simulink model "mpc1"  (R2018a)
settings: Solver=FixedStepAuto  StartTime=0.0  StopTime=inf  RelTol=1e-3  EnableMultiTasking=on
libraries: arduinolib x4, simulink x2, mpclib x1
settings Model: SimulationMode=external  ExtModeTrigDuration=2  Creator=stayn  LastModifiedBy=stayn
settings OptimizationCC: EnhancedBackFolding=on  PassReuseOutputArgsAs=Individual arguments  MaxStackSize=64  OptimizeBlockOrder=speed  DifferentSizesBufferReuse=on  OptimizationCustomize=off
settings DebuggingCC: ParameterTunabilityLossMsg=error
settings HardwareCC: ProdBitPerInt=16  ProdBitPerPointer=16  ProdBitPerSizeT=16  ProdBitPerPtrDiffT=16  ProdLargestAtomicFloat=None  ProdWordSize=8  ProdHWDeviceType=Atmel->AVR
settings SFSimCC: MATLABDynamicMemAlloc=off
settings RTWCC: SystemTargetFile=ert.tlc  HardwareBoard=Arduino Mega 2560  TLCOptions=-aInlineSetEventsForThisBaseRateFcn=TLC_FALSE -aSuppressMultiTaskScheduler=TLC_FALSE -aRateBasedStepFcn=1  TemplateMakefile=ert_default_tmf  GenerateReport=on  Toolchain=Arduino AVR  BuildConfiguration=Faster Runs  IncludeHyperlinkInReport=on  LaunchReport=on  GenerateTraceInfo=on  GenerateTraceReport=on  GenerateTraceReportSl=on  GenerateTraceReportSf=on  GenerateTraceReportEml=on
settings CodeAppCC: ForceParamTrailComments=on  IgnoreCustomStorageClasses=off  OperatorAnnotations=on  SimulinkDataObjDesc=on  SFDataObjDesc=on  InsertBlockDesc=on
settings ERTTargetCC: SupportContinuousTime=on  SupportVariableSizeSignals=on

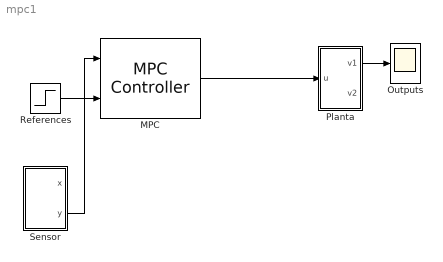
== system mpc1 ==
  MPC : mpclib/MPC Controller  SCDEnableBlockLinearizationSpecification=on  mpcobj=mpc1_C  is_multiple=0  enable_value=0  return_u0=off  updateMPCinCallerWorkspace=on  ref_from_ws=off  ref_signal_name=[]  ref_preview=off  md_from_ws=off  md_signal_name=[]  md_preview=off  from_project=off  project_file=MPCtask.mat  md_inport=off  mv_inport=off  cost_outport=off  return_sequence=off  return_qpstatus=off  return_state=off  state_inport=off  lims_inport=off  cc_inport=off  ywt_inport=off  is_designfromscratch=0  uwt_inport=off  duwt_inport=off  rhoeps_inport=off  uref_inport=off  n_ts=0.1  n_p=10  n_mv=2  n_md=0  n_ud=0  n_mo=2  n_uo=0  BlockDataType=double  SampleTimeInherited=off  switch_inport=off
  Outputs : Scope
  Planta : Subsystem
  References : Step  Before=[0;0]  After=[1;0]
  Sensor : Subsystem
  wires:
  References/1 -> MPC/2
  Planta/1(v1) -> Outputs/1
  MPC/1 -> Planta/1(u)
  Sensor/2(y) -> MPC/1

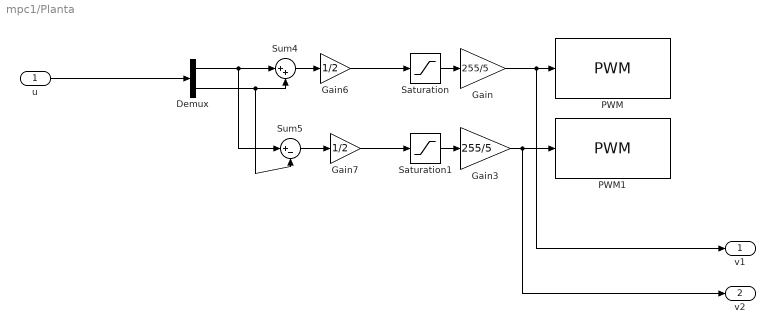
== system mpc1/Planta ==
  u : Inport
  Demux : Demux  Outputs=2
  Gain : Gain  Gain=255/5
  Gain3 : Gain  Gain=255/5
  Gain6 : Gain  Gain=1/2
  Gain7 : Gain  Gain=1/2
  PWM : arduinolib/PWM  pinNumber=9  EnableInputFrequency=off  InitialFrequency=2000  InitialDutyCycle=0  NotificationType=None  blockPlatform=arduino
  PWM1 : arduinolib/PWM  pinNumber=8  EnableInputFrequency=off  InitialFrequency=2000  InitialDutyCycle=0  NotificationType=None  blockPlatform=arduino
  Saturation : Saturate  UpperLimit=5  LowerLimit=0
  Saturation1 : Saturate  UpperLimit=5  LowerLimit=0
  Sum4 : Sum  Inputs=|++
  Sum5 : Sum  Inputs=|+-
  v1 : Outport
  "v2 " : Outport  Port=2
  wires:
  Sum4/1 -> Gain6/1
  Demux/1 -> Sum5/1, Sum4/1
  Saturation1/1 -> Gain3/1
  Gain7/1 -> Saturation1/1
  Demux/2 -> Sum5/2, Sum4/2
  Gain/1 -> PWM/1, v1/1
  Saturation/1 -> Gain/1
  Gain6/1 -> Saturation/1
  Gain3/1 -> PWM1/1, "v2 "/1
  Sum5/1 -> Gain7/1
  u/1 -> Demux/1

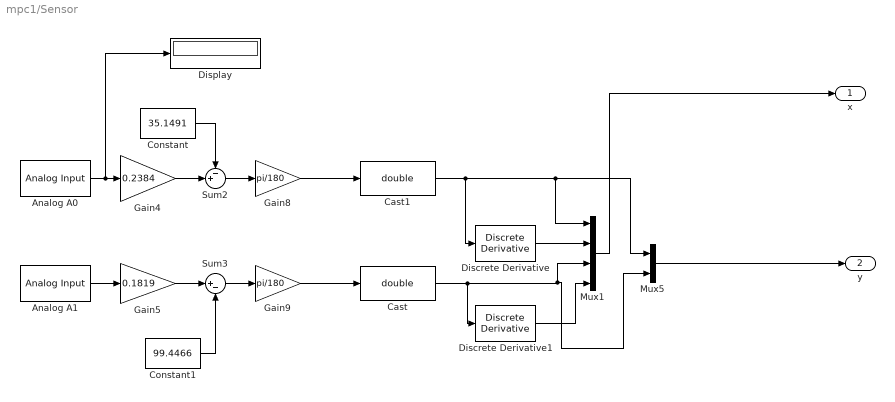
== system mpc1/Sensor ==
  Analog A0 : arduinolib/Analog Input  pinNumber=0  ReadResultsOnly=off  ConversionTriggerSource=Software  ExternalTriggerType=uint32(0)  OutputDataType=uint16  EnableConversionCompleteNotify=off  EnableOuputStatus=off  SampleTime=-1  blockPlatform=arduino
  Analog A1 : arduinolib/Analog Input  pinNumber=1  ReadResultsOnly=off  ConversionTriggerSource=Software  ExternalTriggerType=uint32(0)  OutputDataType=uint16  EnableConversionCompleteNotify=off  EnableOuputStatus=off  SampleTime=-1  blockPlatform=arduino
  Cast : DataTypeConversion  OutDataTypeStr=double
  Cast1 : DataTypeConversion  OutDataTypeStr=double
  Constant : Constant  Value=35.1491
  Constant1 : Constant  Value=99.4466
  Discrete Derivative : simulink/Discrete/Discrete Derivative  gainval=1.0  ICPrevScaledInput=0.0  OutMin=[]  OutMax=[]  OutDataType=fixdt(1, 16)  OutScaling=2^-10  DoSatur=off
  Discrete Derivative1 : simulink/Discrete/Discrete Derivative  gainval=1.0  ICPrevScaledInput=0.0  OutMin=[]  OutMax=[]  OutDataType=fixdt(1, 16)  OutScaling=2^-10  DoSatur=off
  Display : Display
  Gain4 : Gain  Gain=0.2384
  Gain5 : Gain  Gain=0.1819
  Gain8 : Gain  Gain=pi/180
  Gain9 : Gain  Gain=pi/180
  Mux1 : Mux
  Mux5 : Mux  Inputs=2
  Sum2 : Sum  Inputs=-+|
  Sum3 : Sum  Inputs=|+-
  "x " : Outport
  y : Outport  Port=2
  wires:
  Mux5/1 -> y/1
  Cast/1 -> Mux5/2, Mux1/3, Discrete Derivative1/1
  Gain4/1 -> Sum2/2
  Cast1/1 -> Discrete Derivative/1, Mux5/1, Mux1/1
  Sum2/1 -> Gain8/1
  Analog A1/1 -> Gain5/1
  Constant/1 -> Sum2/1
  Constant1/1 -> Sum3/2
  Discrete Derivative1/1 -> Mux1/4
  Mux1/1 -> "x "/1
  Analog A0/1 -> Display/1, Gain4/1
  Discrete Derivative/1 -> Mux1/2
  Gain9/1 -> Cast/1
  Sum3/1 -> Gain9/1
  Gain5/1 -> Sum3/1
  Gain8/1 -> Cast1/1
